simulink library "Lib_Turbo_Splitter_TMATS"  (R2019b)
settings: Solver=ode45  StartTime=0.0  StopTime=10.0  RelTol=1e-3  EnableMultiTasking=on
Description:
  | Thomas Modules
settings Model: Creator=jwchapm2  LastModifiedBy=bhisma
settings DataIOCC: LimitDataPoints=on  SaveFormat=Array  ReturnWorkspaceOutputs=off
settings OptimizationCC: ExpressionDepthLimit=2147483647  LifeSpan=inf
settings DebuggingCC: UnderspecifiedInitializationDetection=Classic  MergeDetectMultiDrivingBlocksExec=none  SolverPrmCheckMsg=warning  StateNameClashWarn=warning  SFUnexpectedBacktrackingDiag=warning  SFNoUnconditionalDefaultTransitionDiag=warning  SFExecutionAtInitializationDiag=none  ArithmeticOperatorsInVariantConditions=warning
settings HardwareCC: ProdBitPerPointer=32  ProdBitPerSizeT=32  ProdBitPerPtrDiffT=32  ProdLargestAtomicFloat=None  ProdIntDivRoundTo=Undefined  ProdEndianess=Unspecified  ProdWordSize=32  ProdHWDeviceType=32-bit Generic
settings ModelReferenceCC: PropagateSignalLabelsOutOfModel=off
settings SFSimCC: SimUseLocalCustomCode=off  CustomCodeUndefinedFunction=UseInterfaceOnly
settings RTWCC: RTWUseLocalCustomCode=off
settings CodeAppCC: StateflowObjectComments=on
settings GRTTargetCC: TargetLangStandard=C89/C90 (ANSI)  GeneratePreprocessorConditionals=Disable all
settings ConfigComp: CovMetricSettings=dw  CovHtmlReporting=on  CovSaveCumulativeToWorkspaceVar=on  CovSaveSingleToWorkspaceVar=on  CovExternalEMLEnable=off

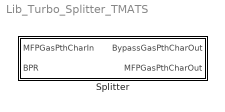
== system Lib_Turbo_Splitter_TMATS ==
  Splitter : Subsystem  mask(T-MATS: Splitter Library Block){}
      mask help: This block simulates the performance of a splitter/bypass using basic flow relationships.
      mask Help: web(which('Turbo_TMATS_Splt.html'),'-helpbrowser')

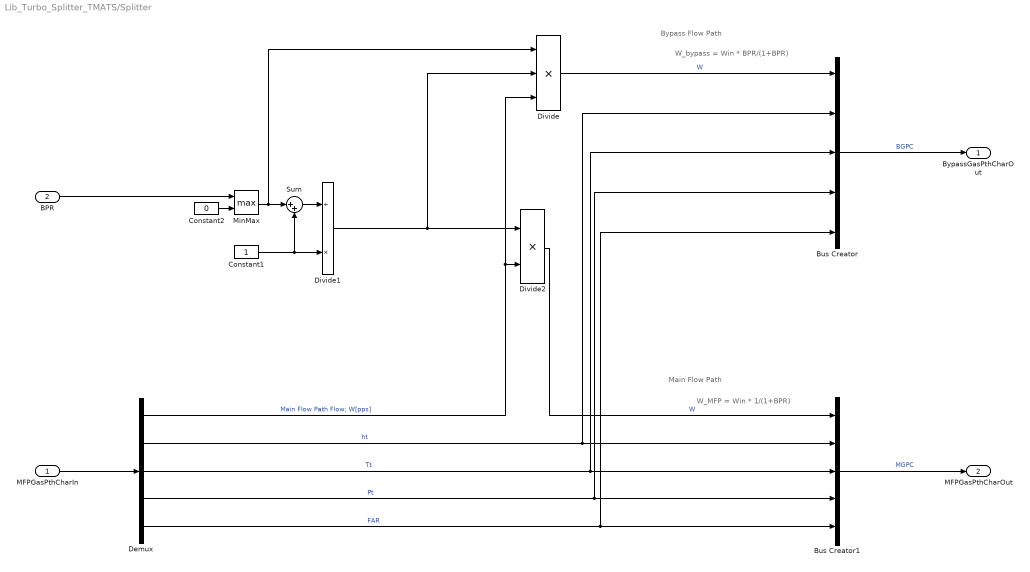
== system Lib_Turbo_Splitter_TMATS/Splitter ==
  note: Main Flow Path
  note: W_bypass = Win * BPR/(1+BPR)
  note: W_MFP = Win * 1/(1+BPR)
  note: Bypass Flow Path
  MFPGasPthCharIn : Inport
  BPR : Inport  Port=2
  Bus Creator : BusCreator  Inputs=5
  Bus Creator1 : BusCreator  Inputs=5
  Constant1 : Constant
  Constant2 : Constant  Value=0
  Demux : Demux  Outputs=5
  Divide : Product  Inputs=***
  Divide1 : Product  Inputs=/*
  Divide2 : Product  Inputs=**
  MinMax : MinMax  Function=max  Inputs=2
  Sum : Sum  Inputs=|++
  BypassGasPthCharOut : Outport
  MFPGasPthCharOut : Outport  Port=2
  wires:
  Bus Creator/1 -> BypassGasPthCharOut/1  "BGPC"
  MFPGasPthCharIn/1 -> Demux/1
  Bus Creator1/1 -> MFPGasPthCharOut/1  "MGPC"
  Constant1/1 -> Divide1/2, Sum/2
  Divide2/1 -> Bus Creator1/1  "W"
  Divide/1 -> Bus Creator/1  "W"
  Demux/5 -> Bus Creator/5, Bus Creator1/5  "FAR"
  Demux/3 -> Bus Creator/3, Bus Creator1/3  "Tt"
  Demux/4 -> Bus Creator/4, Bus Creator1/4  "Pt"
  Sum/1 -> Divide1/1
  Demux/1 -> Divide/3, Divide2/2  "Main Flow Path Flow; W[pps]"
  Divide1/1 -> Divide/2, Divide2/1
  Demux/2 -> Bus Creator/2, Bus Creator1/2  "ht"
  MinMax/1 -> Divide/1, Sum/1
  Constant2/1 -> MinMax/2
  BPR/1 -> MinMax/1
